simulink model "ex3_sim1m"  (R2022b)
settings: Solver=ode45  StartTime=0.0  StopTime=6  MaxStep=0.001  RelTol=1e-3
undefined symbols (not defined in the file): d, mot, pid, q, r, umax
settings Model: Creator=loren  LastModifiedBy=loren
settings DataIOCC: ReturnWorkspaceOutputs=off

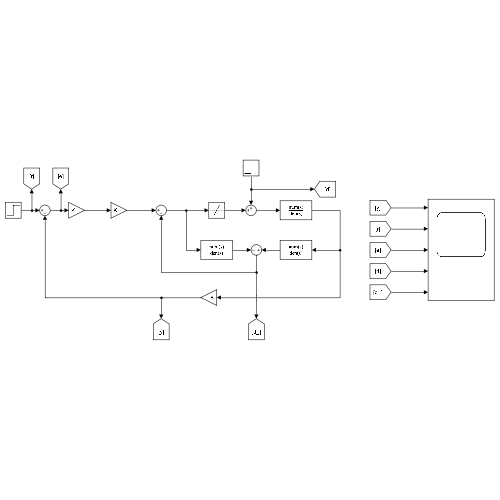
[thumbnail: Simulink's stored preview of the top-level diagram]
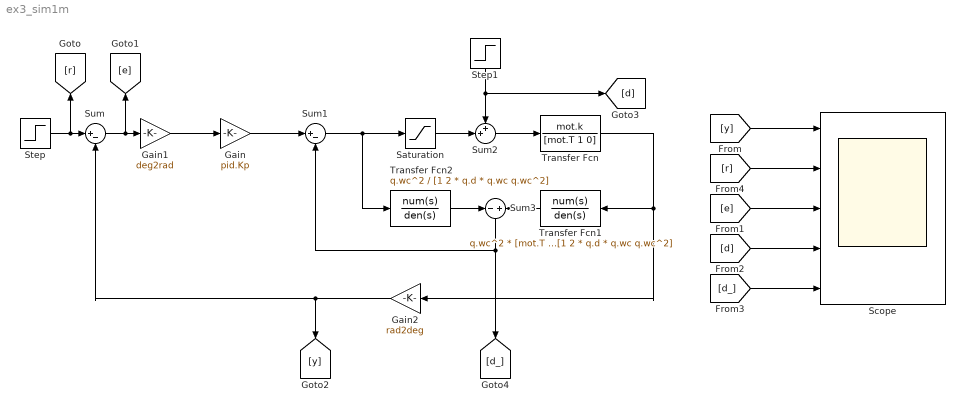
== system ex3_sim1m ==
  Gain : Gain  Gain=pid.Kp
  Gain1 : Gain  Gain=deg2rad
  Gain2 : Gain  Gain=rad2deg
  Saturation : Saturate  UpperLimit=umax  LowerLimit=-umax
  Scope : Scope  NumInputPorts=5
  Step : Step  Time=r.t  After=r.A  SampleTime=0
  Step1 : Step  Time=d.t  After=d.A  SampleTime=0
  Sum : Sum  Inputs=|+-
  Sum1 : Sum  Inputs=|+-
  Sum2 : Sum  Inputs=++|
  Sum3 : Sum  Inputs=-|+
  Transfer Fcn : TransferFcn  Numerator=mot.k  Denominator=[mot.T 1 0]
  Transfer Fcn1 : TransferFcn  Numerator=q.wc^2 * [mot.T 1 0]  Denominator=mot.k * [1 2 * q.d * q.wc q.wc^2]
  Transfer Fcn2 : TransferFcn  Numerator=q.wc^2  Denominator=[1 2 * q.d * q.wc q.wc^2]
  wires:
  Sum/1 -> [e], Gain1/1
  Gain/1 -> Sum1/1
  Sum1/1 -> Transfer Fcn2/1, Saturation/1
  Saturation/1 -> Sum2/2
  Sum2/1 -> Transfer Fcn/1
  Transfer Fcn/1 -> Gain2/1, Transfer Fcn1/1
  Transfer Fcn2/1 -> Sum3/1
  Transfer Fcn1/1 -> Sum3/2
  Sum3/1 -> [d_], Sum1/2
  Gain1/1 -> Gain/1
  Gain2/1 -> [y], Sum/2
  Step1/1 -> [d], Sum2/1
  Step/1 -> [r], Sum/1
  [d_] -> Scope/5
  [d] -> Scope/4
  [e] -> Scope/3
  [r] -> Scope/2
  [y] -> Scope/1
